simulink model "AP_Regelung_Test"  (R2020a)
settings: Solver=VariableStepAuto  StartTime=0.0  StopTime=10  FixedStep=0.001  MaxStep=0.01  RelTol=1e-3
undefined symbols (not defined in the file or in its folder): simparams
settings Model: Creator=Tobias  LastModifiedBy=Tobias
settings SolverCC: ZeroCrossAlgorithm=Adaptive
settings DebuggingCC: IgnoredZcDiagnostic=none

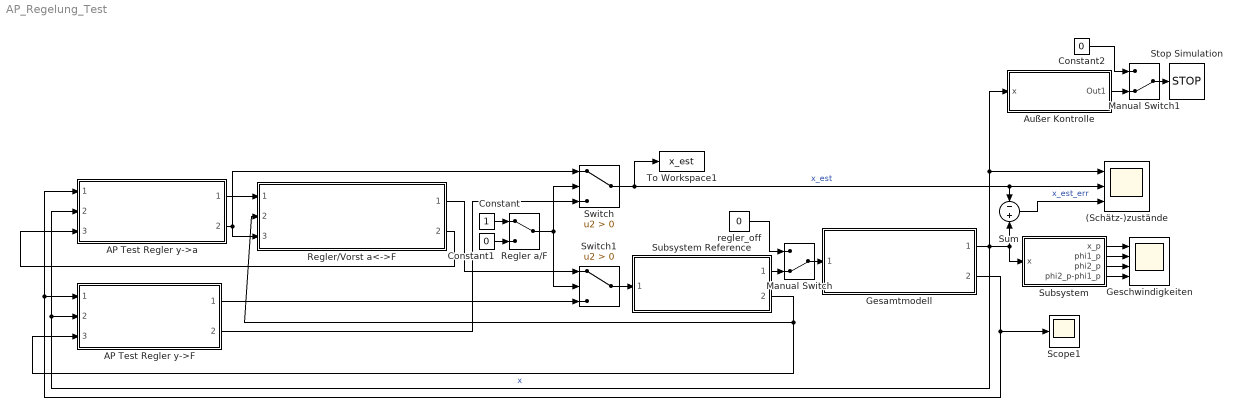
== system AP_Regelung_Test ==
  (Schätz-)zustände : Scope  NumInputPorts=3
  AP Test Regler y->F : Subsystem  ReferencedSubsystem=APRegler  AP=simparams.AP  RegData=simparams.APRegDataF
  AP Test Regler y->a : Subsystem  ReferencedSubsystem=APRegler  AP=simparams.AP  RegData=simparams.APRegDataA
  Außer Kontrolle : Subsystem
  Constant : Constant
  Constant1 : Constant  Value=0
  Constant2 : Constant  Value=0
  Gesamtmodell : Subsystem  ReferencedSubsystem=Gesamtmodell  ModellParameter=simparams.gesamtmodell
  Geschwindigkeiten : Scope  NumInputPorts=4
  Manual Switch : ManualSwitch  CurrentSetting=0
  Manual Switch1 : ManualSwitch  CurrentSetting=0
  Regler a/F : ManualSwitch
  Regler/Vorst a<->F : Subsystem  ReferencedSubsystem=Vorsteuerung_Fa_avRegler  K_p_v=simparams.kpv  a_max=simparams.gesamtmodell.motor.Fmax/simparams.gesamtmodell.schlittenpendel.m0  regler=simparams.regler
  Scope1 : Scope
  Stop Simulation : Stop
  Subsystem : Subsystem
  Subsystem Reference : Subsystem  ReferencedSubsystem=MotorVorsteuerung  MotorGain=simparams.gesamtmodell.motor.staticGain  Umax=simparams.gesamtmodell.motor.Umax_in
  Sum : Sum  Inputs=-+
  Switch : Switch  Criteria=u2 > Threshold
  Switch1 : Switch  Criteria=u2 > Threshold
  To Workspace1 : ToWorkspace  VariableName=x_est  SaveFormat=Timeseries  SampleTime=simparams.tows_ts
  regler_off : Constant  Value=0
  wires:
  AP Test Regler y->F/1 -> Switch1/3
  Gesamtmodell/1 -> (Schätz-)zustände/1, Außer Kontrolle/1(x), Subsystem/1(x), Sum/2, AP Test Regler y->a/2, AP Test Regler y->F/2  "x"
  Switch/1 -> To Workspace1/1, (Schätz-)zustände/2, Sum/1  "x_est"
  Sum/1 -> (Schätz-)zustände/3  "x_est_err"
  Subsystem Reference/1 -> Manual Switch/2
  Manual Switch/1 -> Gesamtmodell/1
  regler_off/1 -> Manual Switch/1
  Switch1/1 -> Subsystem Reference/1
  AP Test Regler y->F/2 -> Switch/3
  Regler/Vorst a<->F/1 -> Switch1/1
  AP Test Regler y->a/2 -> Regler/Vorst a<->F/3, Switch/1
  Regler a/F/1 -> Switch1/2, Switch/2
  Constant/1 -> Regler a/F/1
  Constant1/1 -> Regler a/F/2
  Subsystem Reference/2 -> AP Test Regler y->F/3, Regler/Vorst a<->F/2
  Constant2/1 -> Manual Switch1/1
  Außer Kontrolle/1(Out1) -> Manual Switch1/2
  Manual Switch1/1 -> Stop Simulation/1
  Gesamtmodell/2 -> AP Test Regler y->a/1, AP Test Regler y->F/1, Scope1/1
  Regler/Vorst a<->F/2 -> AP Test Regler y->a/3
  AP Test Regler y->a/1 -> Regler/Vorst a<->F/1
  Subsystem/1(x_p) -> Geschwindigkeiten/1
  Subsystem/2(phi1_p) -> Geschwindigkeiten/2
  Subsystem/3(phi2_p) -> Geschwindigkeiten/3
  Subsystem/4(phi2_p-phi1_p) -> Geschwindigkeiten/4

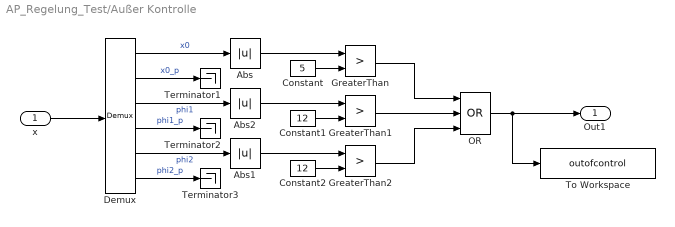
== system AP_Regelung_Test/Außer Kontrolle ==
  x : Inport
  Abs : Abs
  Abs1 : Abs
  Abs2 : Abs
  Constant : Constant  Value=5
  Constant1 : Constant  Value=12
  Constant2 : Constant  Value=12
  Demux : Demux  Outputs=6
  GreaterThan : RelationalOperator  Operator=>  OutDataTypeStr=boolean  RndMeth=Simplest
  GreaterThan1 : RelationalOperator  Operator=>  OutDataTypeStr=boolean  RndMeth=Simplest
  GreaterThan2 : RelationalOperator  Operator=>  OutDataTypeStr=boolean  RndMeth=Simplest
  OR : Logic  Operator=OR  Inputs=3  IconShape=distinctive  AllPortsSameDT=off  OutDataTypeStr=boolean
  Terminator1 : Terminator
  Terminator2 : Terminator
  Terminator3 : Terminator
  To Workspace : ToWorkspace  VariableName=outofcontrol  SaveFormat=Timeseries  SampleTime=-1
  Out1 : Outport
  wires:
  Constant/1 -> GreaterThan/2
  Demux/5 -> Abs1/1  "phi2"
  OR/1 -> To Workspace/1, Out1/1
  Demux/6 -> Terminator3/1  "phi2_p"
  Demux/4 -> Terminator2/1  "phi1_p"
  Abs2/1 -> GreaterThan1/1
  Abs/1 -> GreaterThan/1
  GreaterThan/1 -> OR/1
  GreaterThan1/1 -> OR/2
  Demux/2 -> Terminator1/1  "x0_p"
  Demux/3 -> Abs2/1  "phi1"
  Abs1/1 -> GreaterThan2/1
  Demux/1 -> Abs/1  "x0"
  GreaterThan2/1 -> OR/3
  Constant1/1 -> GreaterThan1/2
  Constant2/1 -> GreaterThan2/2
  x/1 -> Demux/1

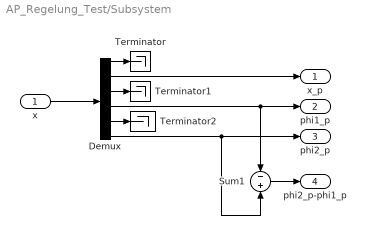
== system AP_Regelung_Test/Subsystem ==
  x : Inport
  Demux : Demux  Outputs=6
  Sum1 : Sum  Inputs=-+
  Terminator : Terminator
  Terminator1 : Terminator
  Terminator2 : Terminator
  x_p : Outport
  phi1_p : Outport  Port=2
  phi2_p : Outport  Port=3
  phi2_p-phi1_p : Outport  Port=4
  wires:
  Demux/4 -> Sum1/1, phi1_p/1
  Demux/2 -> x_p/1
  Demux/5 -> Terminator2/1
  x/1 -> Demux/1
  Demux/3 -> Terminator1/1
  Sum1/1 -> phi2_p-phi1_p/1
  Demux/1 -> Terminator/1
  Demux/6 -> Sum1/2, phi2_p/1
